simulink model "sample_init_func"  (R2019b)
settings: Solver=FixedStepAuto  StartTime=0.0  StopTime=10.0  RelTol=1e-3
settings Model: Creator=N196212  LastModifiedBy=N196212
settings OptimizationCC: DefaultParameterBehavior=Inlined  EnhancedBackFolding=on  PassReuseOutputArgsAs=Individual arguments  ZeroExternalMemoryAtStartup=off  ZeroInternalMemoryAtStartup=off  OptimizeBlockOrder=speed  DifferentSizesBufferReuse=on  OptimizationCustomize=off  EfficientTunableParamExpr=on
settings DebuggingCC: ParameterTunabilityLossMsg=error
settings SFSimCC: MATLABDynamicMemAlloc=off
settings RTWCC: SystemTargetFile=ert.tlc  GenCodeOnly=on  TemplateMakefile=ert_default_tmf  GenerateReport=on  IncludeHyperlinkInReport=on  LaunchReport=on  GenerateTraceInfo=on  GenerateTraceReport=on  GenerateTraceReportSl=on  GenerateTraceReportSf=on  GenerateTraceReportEml=on
settings CodeAppCC: ForceParamTrailComments=on  IgnoreCustomStorageClasses=off  OperatorAnnotations=on  SimulinkDataObjDesc=on  SFDataObjDesc=on  InsertBlockDesc=on
settings ERTTargetCC: TargetLangStandard=C99 (ISO)  GenerateSampleERTMain=on  InlinedParameterPlacement=NonHierarchical  ERTCustomFileTemplate=example_file_process.tlc

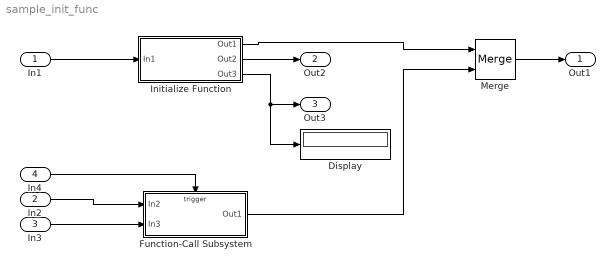
== system sample_init_func ==
  In1 : Inport
  In2 : Inport  Port=2
  In3 : Inport  Port=3
  In4 : Inport  Port=4  OutputFunctionCall=on
  Display : Display
  Function-Call Subsystem : Subsystem  TreatAsAtomicUnit=on
  Initialize Function : Subsystem  TreatAsAtomicUnit=on
  Merge : Merge
  Out1 : Outport
  Out2 : Outport  Port=2
  Out3 : Outport  Port=3
  wires:
  In1/1 -> Initialize Function/1(In1)
  Initialize Function/2(Out2) -> Out2/1
  Merge/1 -> Out1/1
  Function-Call Subsystem/1(Out1) -> Merge/2
  In4/1 -> Function-Call Subsystem/Trigger
  In3/1 -> Function-Call Subsystem/2(In3)
  In2/1 -> Function-Call Subsystem/1(In2)
  Initialize Function/1(Out1) -> Merge/1
  Initialize Function/3(Out3) -> Display/1, Out3/1

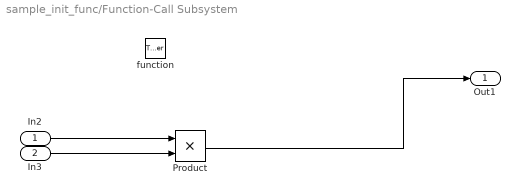
== system sample_init_func/Function-Call Subsystem ==
  In2 : Inport
  In3 : Inport  Port=2
  function : TriggerPort  TriggerType=function-call  VariantControl=Variant
  Product : Product  OutDataTypeStr=uint16
  Out1 : Outport  OutDataTypeStr=uint16
  wires:
  In2/1 -> Product/1
  Product/1 -> Out1/1
  In3/1 -> Product/2

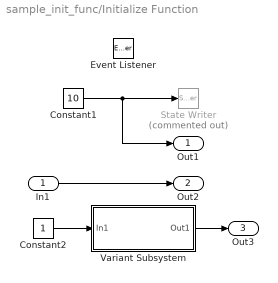
== system sample_init_func/Initialize Function ==
  In1 : Inport
  Constant1 : Constant  Value=10  OutDataTypeStr=uint16
  Constant2 : Constant  OutDataTypeStr=uint8
  Event Listener : EventListener  DisableCoverage=on  EventName=reset  Variant=on
      settings: GeneratePreprocessorConditionals=on
  State Writer : StateWriter  Commented=on
  Variant Subsystem : Subsystem  Variant=on
      settings: GeneratePreprocessorConditionals=on
  Out1 : Outport  OutDataTypeStr=uint16
  Out2 : Outport  Port=2
  Out3 : Outport  Port=3
  wires:
  Constant1/1 -> Out1/1, State Writer/1
  In1/1 -> Out2/1
  Constant2/1 -> Variant Subsystem/1(In1)
  Variant Subsystem/1(Out1) -> Out3/1

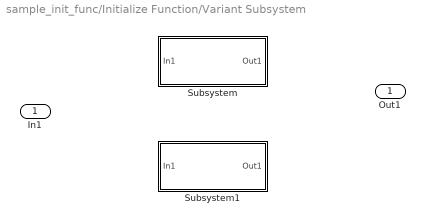
== system sample_init_func/Initialize Function/Variant Subsystem ==
  In1 : Inport
  Subsystem : Subsystem  TreatAsAtomicUnit=on  VariantControl=VariantSub
  Subsystem1 : Subsystem  TreatAsAtomicUnit=on  VariantControl=VariantSub2
  Out1 : Outport

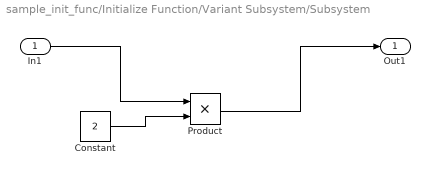
== system sample_init_func/Initialize Function/Variant Subsystem/Subsystem ==
  In1 : Inport
  Constant : Constant  Value=2
  Product : Product
  Out1 : Outport
  wires:
  Constant/1 -> Product/2
  In1/1 -> Product/1
  Product/1 -> Out1/1

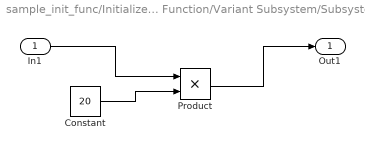
== system sample_init_func/Initialize Function/Variant Subsystem/Subsystem1 ==
  In1 : Inport
  Constant : Constant  Value=20
  Product : Product
  Out1 : Outport
  wires:
  Constant/1 -> Product/2
  In1/1 -> Product/1
  Product/1 -> Out1/1
